simulink model "modele"  (R2018b)
settings: Solver=VariableStepAuto  StartTime=0.0  StopTime=10.0  RelTol=1e-3
values from neighbouring files (symbols this model uses):
  Cb = 9.97*(10^(-2))    (= 0.0997)    [parametres_cubli.m]
  Cw = 2.95e-5    (= 2.95e-05)    [parametres_cubli.m]
  g = 9.81    [parametres_cubli.m]
  Ib = 3.43*(10^(-3))    (= 0.00343)    [parametres_cubli.m]
  Iw = 2.63*(10^(-4))    (= 0.000263)    [parametres_cubli.m]
  Ki = 25.1*0.001    (= 0.0251)    [parametres_cubli.m]
  l = 9.65*0.01    (= 0.0965)    [parametres_cubli.m]
  lb = 10.35*0.01    (= 0.1035)    [parametres_cubli.m]
  mb = 0.43    [parametres_cubli.m]
  mw = 0.096    [parametres_cubli.m]
  Theta_b_ini = 0.125    [parametres_cubli.m]
undefined symbols (not defined in the file or in its folder): K, K3, sigbuilder_block
libraries: c2837xDlib x1
settings Model: Creator=ntest557  LastModifiedBy=ntest557

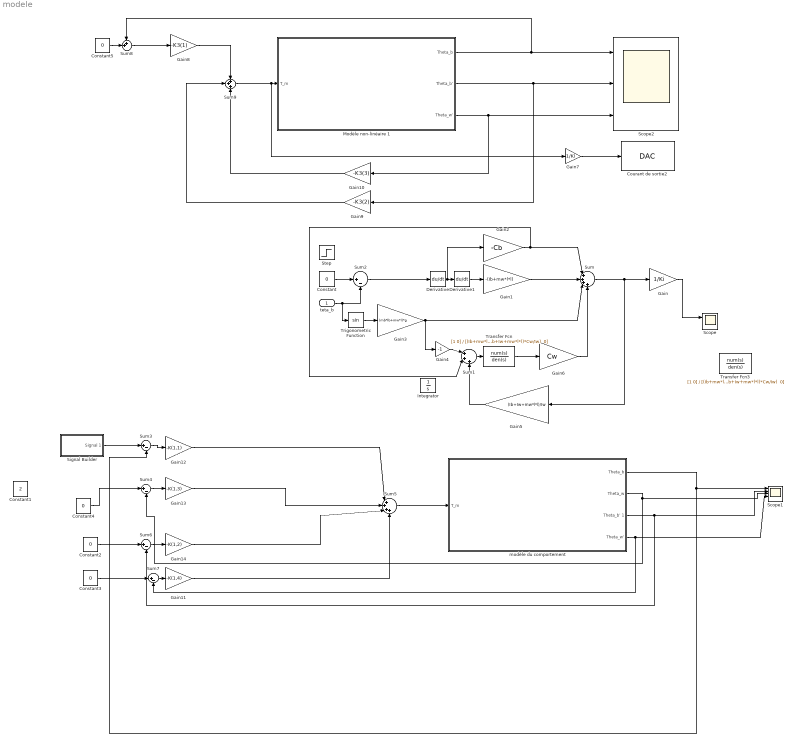
== system modele ==
  teta_b : Inport
  Constant{,2..5} (5 alike) : Constant  Value=0
  Constant1 : Constant  Value=2
  Courant de sortie2 : c2837xDlib/DAC  channel=A  saturate=off
      settings: SourceProductName=Embedded Coder Support Package for Texas Instruments C2000 Processors  SourceProductBaseCode=TIC2000
  Derivative : Derivative
  Derivative1 : Derivative
  Gain : Gain  Gain=1/Ki
  Gain1 : Gain  Gain=-(Ib+mw*l*l)
  Gain10 : Gain  Gain=-K3(3)
  Gain11 : Gain  Gain=-K(1,4)
  Gain12 : Gain  Gain=-K(1,1)
  Gain13 : Gain  Gain=-K(1,3)
  Gain14 : Gain  Gain=-K(1,2)
  Gain2 : Gain  Gain=-Cb
  Gain3 : Gain  Gain=(mb*lb+mw*l)*g
  Gain4 : Gain  Gain=-1
  Gain5 : Gain  Gain=(Ib+Iw+mw*l*l)/Iw
  Gain6 : Gain  Gain=Cw
  Gain7 : Gain  Gain=1/Ki
  Gain8 : Gain  Gain=-K3(1)
  Gain9 : Gain  Gain=-K3(2)
  Integrator : Integrator
  Modèle non-linéaire 1 : Subsystem
  Scope : Scope  NumInputPorts=2
  Scope1 : Scope  NumInputPorts=5
  Scope2 : Scope  NumInputPorts=3
  Signal Builder : Subsystem  Tag=STV Subsys  LoadFcn=sigbuilder_block('load');  StartFcn=sigbuilder_block('start');  StopFcn=sigbuilder_block('stop');  ClipboardFcn=sigbuilder_block('clipboard');  mask(Sigbuilder block){tuvar=[0:10]}
      mask help: Simulink:masks:SigbuilderBlock_MD
      mask init:
      | if ~strcmp(get_param(bdroot(gcbh),'SimulationStatus'),'stopped') tuvar = sigbuilder_block('maskInit'); end
      settings: CopyFcn=sigbuilder_block('copy');  DeleteFcn=sigbuilder_block('delete');  ModelCloseFcn=sigbuilder_block('modelClose');  PreSaveFcn=sigbuilder_block('preSave');  PauseFcn=sigbuilder_block('pause');  ContinueFcn=sigbuilder_block('continue');  NameChangeFcn=sigbuilder_block('namechange');  OpenFcn=sigbuilder_block('open',[437.6 199.2 550.4 400 ]);  CloseFcn=sigbuilder_block('close');
      mask Display: plot(0, 0, 100, 100,[2, 2, 32, 32, 2], [68, 8, 8, 68, 68],[32, 2], [38, 38], [32, 19, 2],[53, 60, 44], [32, 17, 17, 2],[16, 16, 31, 31]);txt = getActiveGroup(gcbh);text(2, 100, txt,'verticalAlignment', 'top');
  Step : Step  SampleTime=0
  Sum : Sum  Inputs=|++++
  Sum1 : Sum  Inputs=|+++
  Sum{2..4,6..7} (5 alike) : Sum  Inputs=|+-
  Sum5 : Sum  Inputs=|++++
  Sum8 : Sum  Inputs=++|
  Sum9 : Sum  Inputs=+++
  Transfer Fcn : TransferFcn  Numerator=[1 0]  Denominator="[(Ib+mw*l*l)  ((Ib+Iw+mw*l*l)*Cw/Iw)  0]"
  Transfer Fcn3 : TransferFcn  Numerator=[1 0]  Denominator="[(Ib+mw*l*l)  ((Ib+Iw+mw*l*l)*Cw/Iw)  0]"
  Trigonometric Function : Trigonometry
  modèle du comportement : Subsystem
  wires:
  Derivative/1 -> Gain2/1, Derivative1/1
  Derivative1/1 -> Gain1/1
  Trigonometric Function/1 -> Gain3/1
  Gain2/1 -> Sum1/2, Sum/1
  Gain1/1 -> Sum/2
  Gain3/1 -> Gain4/1, Sum/3
  Sum/1 -> Gain5/1, Gain/1
  Gain4/1 -> Sum1/1
  Gain5/1 -> Sum1/3
  Sum1/1 -> Transfer Fcn/1
  Transfer Fcn/1 -> Gain6/1
  Gain6/1 -> Sum/4
  Sum2/1 -> Derivative/1
  Gain/1 -> Scope/1
  Constant/1 -> Sum2/1
  teta_b/1 -> Trigonometric Function/1, Sum2/2
  Sum5/1 -> modèle du comportement/1("T_m ")
  Gain12/1 -> Sum5/1
  modèle du comportement/3(Theta_b' 1) -> Sum6/2, Scope1/2
  modèle du comportement/4(Theta_w') -> Scope1/4, Sum7/2
  modèle du comportement/2(Theta_w) -> Sum4/2, Scope1/3
  modèle du comportement/1("Theta_b ") -> Scope1/1, Sum3/2
  Sum3/1 -> Gain12/1
  Signal Builder/1(Signal 1) -> Sum3/1
  Sum6/1 -> Gain14/1
  Sum7/1 -> Gain11/1
  Sum4/1 -> Gain13/1
  Constant4/1 -> Sum4/1
  Constant2/1 -> Sum6/1
  Constant3/1 -> Sum7/1
  Gain14/1 -> Sum5/3
  Gain13/1 -> Sum5/2
  Gain11/1 -> Sum5/4
  Sum8/1 -> Gain8/1
  Gain8/1 -> Sum9/1
  Constant5/1 -> Sum8/2
  Modèle non-linéaire 1/2("Theta_b' ") -> Scope2/2, Gain9/1
  Gain9/1 -> Sum9/2
  Modèle non-linéaire 1/3(Theta_w') -> Scope2/3, Gain10/1
  Gain10/1 -> Sum9/3
  Sum9/1 -> Gain7/1, Modèle non-linéaire 1/1("T_m ")
  Gain7/1 -> Courant de sortie2/1
  Modèle non-linéaire 1/1("Theta_b ") -> Scope2/1, Sum8/1

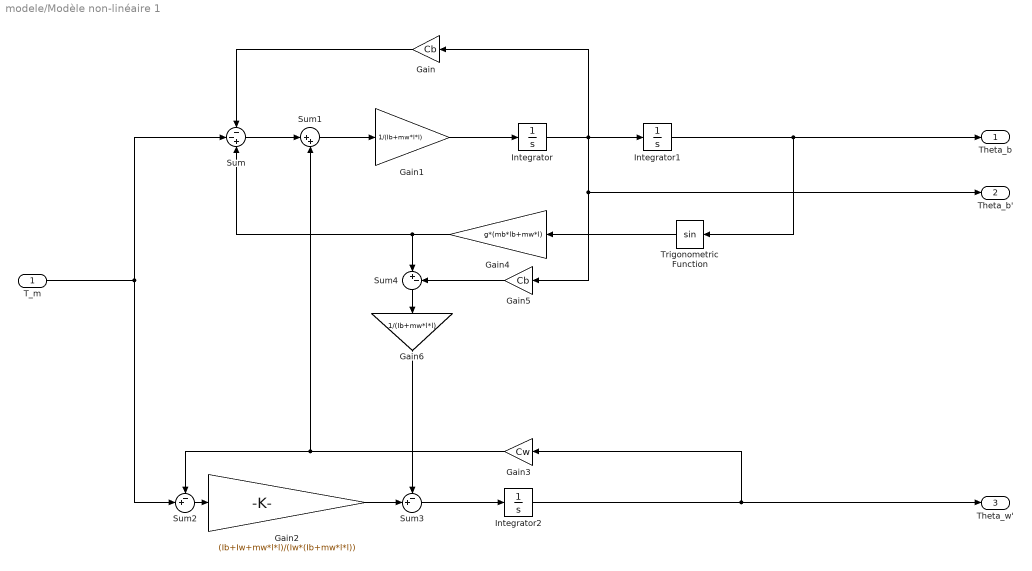
== system modele/Modèle non-linéaire 1 ==
  "T_m " : Inport
  Gain : Gain  Gain=Cb
  Gain1 : Gain  Gain=1/(Ib+mw*l*l)
  Gain2 : Gain  Gain=(Ib+Iw+mw*l*l)/(Iw*(Ib+mw*l*l))
  Gain3 : Gain  Gain=Cw
  Gain4 : Gain  Gain=g*(mb*lb+mw*l)
  Gain5 : Gain  Gain=Cb
  Gain6 : Gain  Gain=1/(Ib+mw*l*l)
  Integrator : Integrator
  Integrator1 : Integrator  InitialCondition=Theta_b_ini
  Integrator2 : Integrator
  Sum : Sum  Inputs=--+
  Sum1 : Sum  Inputs=|++
  Sum2 : Sum  Inputs=-+|
  Sum3 : Sum  Inputs=-+|
  Sum4 : Sum  Inputs=|+-
  Trigonometric Function : Trigonometry
  "Theta_b " : Outport
  "Theta_b' " : Outport  Port=2
  Theta_w' : Outport  Port=3
  wires:
  Gain/1 -> Sum/1
  Sum/1 -> Sum1/1
  Sum1/1 -> Gain1/1
  Gain1/1 -> Integrator/1
  Integrator/1 -> Integrator1/1, Gain5/1, "Theta_b' "/1, Gain/1
  "T_m "/1 -> Sum2/2, Sum/2
  Integrator1/1 -> Trigonometric Function/1, "Theta_b "/1
  Sum2/1 -> Gain2/1
  Gain2/1 -> Sum3/2
  Sum3/1 -> Integrator2/1
  Integrator2/1 -> Gain3/1, Theta_w'/1
  Gain3/1 -> Sum1/2, Sum2/1
  Trigonometric Function/1 -> Gain4/1
  Gain4/1 -> Sum/3, Sum4/1
  Sum4/1 -> Gain6/1
  Gain5/1 -> Sum4/2
  Gain6/1 -> Sum3/1

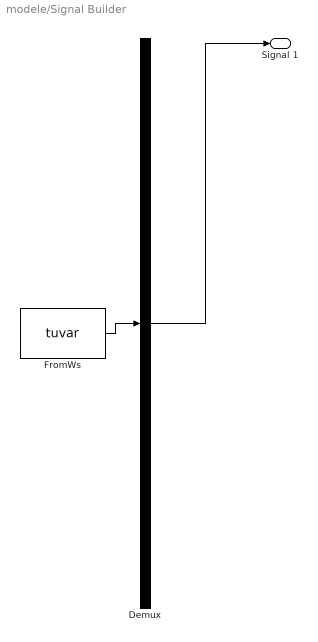
== system modele/Signal Builder ==
  Demux : Demux  Tag=STV Demux  Outputs=1
  FromWs : FromWorkspace  Tag=STV FromWs  VariableName=tuvar  SampleTime=0
      SigBuilderData=|
      | common.afterFinalStr = 'Extrapolate'
      | common.sampleTime = 0
      | dataSet.timeRange = [0 10]
      | dataSet.name = 'Group 1'
      | sbobj.Groups.Name = 'Group 1'
      | sbobj.Groups.Signals.Name = 'Signal 1'
      | sbobj.Groups.Signals.XData = [0 4 4 4.5 4.5 10]
      | sbobj.Groups.Signals.YData = [0 0 0.1 0.1 0 0]
  Signal 1 : Outport  Tag=STV Outport
  wires:
  Demux/1 -> Signal 1/1
  FromWs/1 -> Demux/1

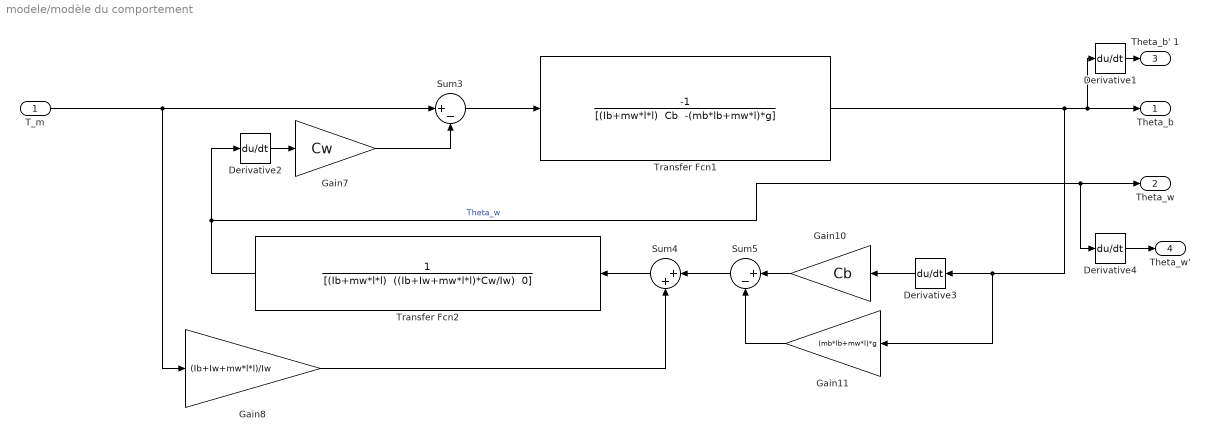
== system modele/modèle du comportement ==
  "T_m " : Inport
  Derivative{1..4} (4 alike) : Derivative
  Gain10 : Gain  Gain=Cb
  Gain11 : Gain  Gain=(mb*lb+mw*l)*g
  Gain7 : Gain  Gain=Cw
  Gain8 : Gain  Gain=(Ib+Iw+mw*l*l)/Iw
  Sum3 : Sum  Inputs=|+-
  Sum4 : Sum  Inputs=|++
  Sum5 : Sum  Inputs=|+-
  Transfer Fcn1 : TransferFcn  Numerator=[-1]  Denominator="[(Ib+mw*l*l)  Cb  -(mb*lb+mw*l)*g]"
  Transfer Fcn2 : TransferFcn  Denominator="[(Ib+mw*l*l)  ((Ib+Iw+mw*l*l)*Cw/Iw)  0]"
  "Theta_b " : Outport
  Theta_w : Outport  Port=2
  Theta_b' 1 : Outport  Port=3
  Theta_w' : Outport  Port=4
  wires:
  Transfer Fcn2/1 -> Derivative4/1, Theta_w/1, Derivative2/1  "Theta_w"
  Gain8/1 -> Sum4/2
  Sum4/1 -> Transfer Fcn2/1
  "T_m "/1 -> Gain8/1, Sum3/1
  Gain10/1 -> Sum5/1
  Derivative2/1 -> Gain7/1
  Sum3/1 -> Transfer Fcn1/1
  Gain7/1 -> Sum3/2
  Derivative3/1 -> Gain10/1
  Sum5/1 -> Sum4/1
  Gain11/1 -> Sum5/2
  Transfer Fcn1/1 -> Derivative3/1, Gain11/1, Derivative1/1, "Theta_b "/1
  Derivative4/1 -> Theta_w'/1
  Derivative1/1 -> Theta_b' 1/1
